simulink model "pendulum"  (R2024b)
settings: Solver=VariableStepAuto  StartTime=0.0  StopTime=10.0  RelTol=1e-3
settings Model: Creator=Botló  LastModifiedBy=Botló

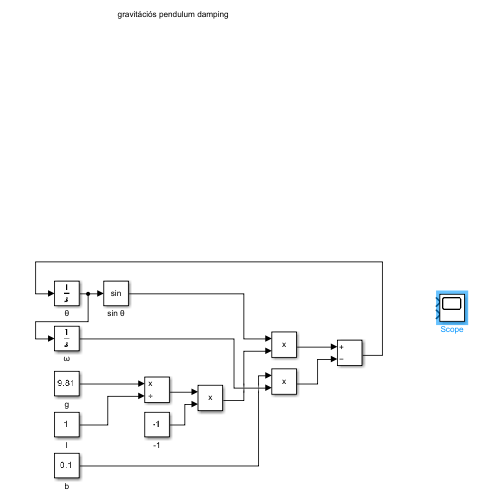
[thumbnail: Simulink's stored preview of the top-level diagram]
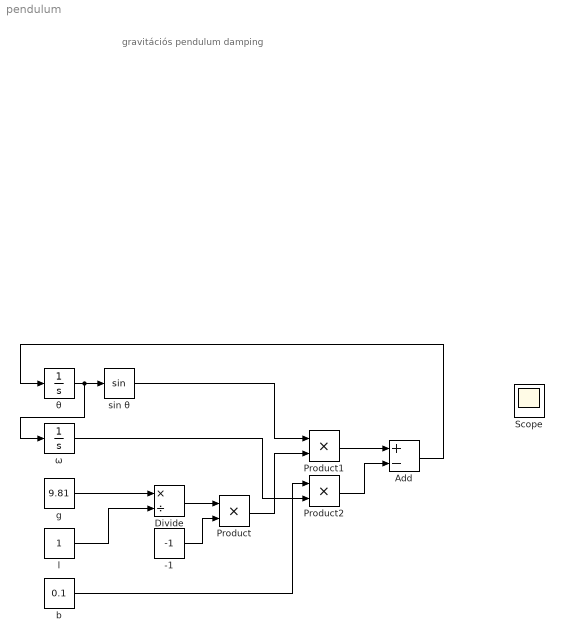
== system pendulum ==
  note: gravitációs pendulum damping
  -1 : Constant  Value=-1
  Add : Sum  Inputs=+-
  Divide : Product  Inputs=*/
  Product : Product
  Product1 : Product
  Product2 : Product
  Scope : Scope  NumInputPorts=2
  b : Constant  Value=0.1
  g : Constant  Value=9.81
  l : Constant
  sin θ : Trigonometry
  θ : Integrator
  ω : Integrator
  wires:
  θ/1 -> ω/1, sin θ/1
  g/1 -> Divide/1
  l/1 -> Divide/2
  Divide/1 -> Product/1
  -1/1 -> Product/2
  sin θ/1 -> Product1/1
  Product/1 -> Product1/2
  Product1/1 -> Add/1
  Product2/1 -> Add/2
  b/1 -> Product2/1
  ω/1 -> Product2/2
  Add/1 -> θ/1
